simulink model "Assignment1_V4"  (R2022b)
settings: Solver=FixedStepAuto  StartTime=0.0  StopTime=10.0  RelTol=1e-3  EnableMultiTasking=on
undefined symbols (not defined in the file or in its folder): A0, A1, D0, D1, D10, D11, D12, D13, D2, D3, D4, D5, D6, D7, D8, D9, PTA0, PTA1, PTA2, PTB2, PTB23, PTB3, PTB9, PTC16, PTC17, PTC2, PTC3, PTC4, PTD0, PTD1, PTD2, PTD3
libraries: frdmk64flib x25, etargetslib x2
settings Model: ExtModeTrigDuration=5  Creator=a laptop  LastModifiedBy=a laptop
settings OptimizationCC: EnhancedBackFolding=on  PassReuseOutputArgsAs=Individual arguments  ZeroExternalMemoryAtStartup=off  ZeroInternalMemoryAtStartup=off  MaxStackSize=64  OptimizeBlockOrder=speed  DifferentSizesBufferReuse=on  OptimizationCustomize=off  EfficientTunableParamExpr=on
settings DebuggingCC: ParameterTunabilityLossMsg=error
settings HardwareCC: ProdBitPerPointer=32  ProdBitPerSizeT=32  ProdBitPerPtrDiffT=32  ProdLargestAtomicInteger=Long  ProdLargestAtomicFloat=Double  ProdWordSize=32  ProdLongLongMode=on  ProdHWDeviceType=ARM Compatible->ARM Cortex
settings SFSimCC: MATLABDynamicMemAlloc=off
settings RTWCC: Description=Embedded Coder  SystemTargetFile=ert.tlc  HardwareBoard=NXP FRDM-K64F  TLCOptions="-aInlineSetEventsForThisBaseRateFcn=TLC_FALSE -aSuppressMultiTaskScheduler=TLC_FALSE  -aRateBasedStepFcn=0"  TemplateMakefile=ert_default_tmf  Toolchain=GNU Tools for ARM Embedded Processors
settings CodeAppCC: ForceParamTrailComments=on  IgnoreCustomStorageClasses=off  OperatorAnnotations=on  SimulinkDataObjDesc=on  SFDataObjDesc=on  InsertBlockDesc=on
settings ERTTargetCC: SupportVariableSizeSignals=on  ExtModeTransport=4  ExtModeMexFile=sendToCommService

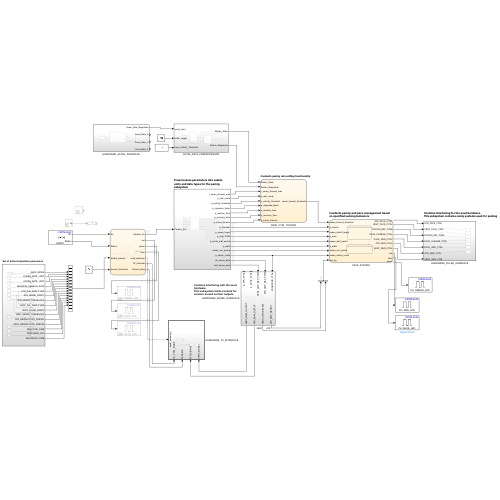
[thumbnail: Simulink's stored preview of the top-level diagram]
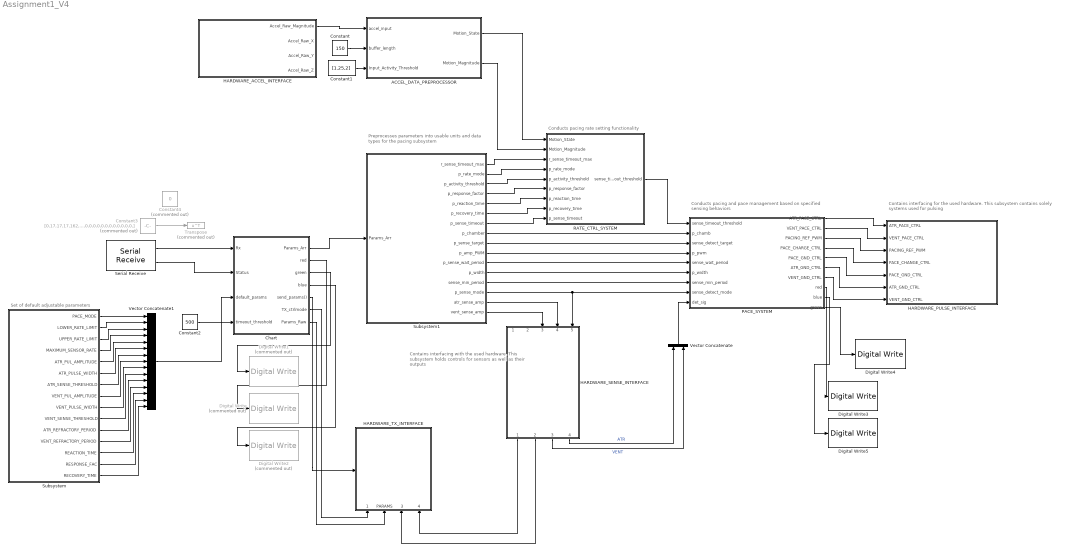
== system Assignment1_V4 ==
  note: Conducts pacing rate setting functionality
  note: Set of default adjustable parameters
  note: Preprocesses parameters into usable units and data types for the pacing subsystem
  note: Contains interfacing with the used hardware.
      | This subsystem holds controls for sensors as well as their outputs
  note: Contains interfacing for the used hardware.
      | This subsystem contains solely systems used for pulsing
  note: Conducts pacing and pace management based on specified sensing behaviors
  ACCEL_DATA_PREPROCESSOR : Subsystem
  Chart : Stateflow chart  TreatAsAtomicUnit=on
      settings: PortSchema="{\"entries\":[{\"content\":{\"sides\":[{\"content\":{\"connectorIds\":[\"In1\",\"In2\",\"In3\",\"In4\"]},\"type\":\"ConnectorPlacement.EquallySpacedRectSide\",\"uuid\":\"320bc760-8283-4f2b-996b-2bacb632d8d9\"},{\"content\":{\"connectorIds\":[\"Out2\",\"Out4\",\"Out5\",\"Out6\",\"Out7\",\"Out3\",\"Out1\"],\"side\":\"RIGHT\"},\"type\":\"ConnectorPlacement.EquallySpacedRectSide\",\"uuid\":\"405a4bb2-50d6-4c0d-b540-a004b1136e76\"},{\"content\":{\"connectorIds\":[],\"side\":\"TOP\"},\"type\":\"ConnectorPlacement.EquallySpacedRectSide\",\"uuid\":\"abc74140-9996-448b-8aab-969529bb67e5\"}]},\"type\":\"ConnectorPlacement.EquallySpacedConnector\",\"uuid\":\"83b64870-f027-44a6-ac9f-b34b790ab38f\"}],\"packageUris\":[\"http://schema.mathworks.com/mf0/Connector/R2020b\"],\"version\":\"1.0\"}"
  Constant : Constant  Value=150
  Constant1 : Constant  Value=[1.25,2]
  Constant2 : Constant  Value=500
  Constant3 : Constant  Commented=on  Value=[0,17,17,17,162,8,0,0,88,2,0,0,176,4,0,0,0,0,0,0,0,0,0,0,0,0,0,0,0,0,0,0,35,0,0,0,10,0,0,0,35,0,0,0,0,0,0,0,128,12,0,0,0,0,0,0,0,0,0,0,0,0,0,0,]  OutDataTypeStr=uint8
  Constant4 : Constant  Commented=on  Value=0  OutDataTypeStr=uint8
  Digital Write : frdmk64flib/Digital Write  Commented=on  Whichpin=RED_LED
  Digital Write1 : frdmk64flib/Digital Write  Commented=on  Whichpin=GREEN_LED
  Digital Write2 : frdmk64flib/Digital Write  Commented=on  Whichpin=BLUE_LED
  Digital Write3 : frdmk64flib/Digital Write  Whichpin=RED_LED
  Digital Write4 : frdmk64flib/Digital Write  Whichpin=GREEN_LED
  Digital Write5 : frdmk64flib/Digital Write  Whichpin=BLUE_LED
  HARDWARE_ACCEL_INTERFACE : Subsystem
  HARDWARE_PULSE_INTERFACE : Subsystem
  HARDWARE_SENSE_INTERFACE : Subsystem
  HARDWARE_TX_INTERFACE : Subsystem
  PACE_SYSTEM : Stateflow chart  TreatAsAtomicUnit=on
      settings: PortSchema="{\"entries\":[{\"content\":{\"sides\":[{\"content\":{\"connectorIds\":[\"In3\",\"In1\",\"In2\",\"In4\",\"In5\",\"In6\",\"In9\",\"In7\",\"In8\"]},\"type\":\"ConnectorPlacement.EquallySpacedRectSide\",\"uuid\":\"7443a3c3-e653-4ca7-8541-eabcfaf454bc\"},{\"content\":{\"connectorIds\":[\"Out1\",\"Out2\",\"Out3\",\"Out4\",\"Out5\",\"Out6\",\"Out7\",\"Out8\",\"Out9\",\"Out10\"],\"side\":\"RIGHT\"},\"type\":\"ConnectorPlacement.EquallySpacedRectSide\",\"uuid\":\"2c63cfa0-dfd9-4a62-91aa-a60ecd75cc2c\"},{\"content\":{\"connectorIds\":[],\"side\":\"TOP\"},\"type\":\"ConnectorPlacement.EquallySpacedRectSide\",\"uuid\":\"5c2dbe0e-7e89-449d-bdd0-c0f7e700edae\"}]},\"type\":\"ConnectorPlacement.EquallySpacedConnector\",\"uuid\":\"602c7a1c-8730-4b31-b945-266bd0371e8b\"}],\"packageUris\":[\"http://schema.mathworks.com/mf0/Connector/R2020b\"],\"version\":\"1.0\"}"
  RATE_CTRL_SYSTEM : Stateflow chart  TreatAsAtomicUnit=on
  Serial Receive : frdmk64flib/Serial Receive  SCIModule=0  Baudrate=uint32(9600)  Parity=None  StopBits=1  HardwareFlowControl=None  ByteOrder=LittleEndian  DataType=uint8  DataLength=64  BlockingMode=off  OutputStatus=on  SampleTime=-1
  Subsystem : Subsystem
  Subsystem1 : Subsystem
  Transpose : Math  Commented=on  Operator=transpose
  Vector Concatenate : Concatenate
  Vector Concatenate1 : Concatenate  NumInputs=15
  wires:
  Serial Receive/2 -> Chart/2(Status)
  RATE_CTRL_SYSTEM/1(sense_timeout_threshold) -> PACE_SYSTEM/3(sense_timeout_threshold)
  Subsystem1/12(p_width) -> PACE_SYSTEM/6(p_width)
  Subsystem/2(LOWER_RATE_LIMIT) -> Vector Concatenate1/2
  Subsystem1/14(p_sense_mode) -> PACE_SYSTEM/7(sense_detect_mode), HARDWARE_SENSE_INTERFACE/5(FRONTEND_CTRL)
  Subsystem1/15(atr_sense_amp) -> HARDWARE_SENSE_INTERFACE/4(ATR_CMP_REF_PWM)
  PACE_SYSTEM/3(PACING_REF_PWM) -> HARDWARE_PULSE_INTERFACE/3(PACING_REF_PWM)
  Chart/6(blue) -> Digital Write2/1
  Chart/5(green) -> Digital Write1/1
  Subsystem1/7(p_sense_timeout) -> RATE_CTRL_SYSTEM/9(p_sense_timeout)
  Constant3/1 -> Transpose/1
  Subsystem1/1(r_sense_timeout_max) -> RATE_CTRL_SYSTEM/3(r_sense_timeout_max)
  Subsystem/13(REACTION_TIME) -> Vector Concatenate1/13
  Subsystem/15(RECOVERY_TIME) -> Vector Concatenate1/15
  HARDWARE_ACCEL_INTERFACE/1(Accel_Raw_Magnitude) -> ACCEL_DATA_PREPROCESSOR/1(accel_input)
  Constant1/1 -> ACCEL_DATA_PREPROCESSOR/3(Input_Activity_Threshold)
  Subsystem/12(VENT_REFRACTORY_PERIOD) -> Vector Concatenate1/12
  Subsystem/10(VENT_SENSE_THRESHOLD) -> Vector Concatenate1/10
  Subsystem1/2(p_rate_mode) -> RATE_CTRL_SYSTEM/4(p_rate_mode)
  Subsystem/6(ATR_PULSE_WIDTH) -> Vector Concatenate1/6
  HARDWARE_SENSE_INTERFACE/2(ATR_RAW_OUTPUT) -> HARDWARE_TX_INTERFACE/3(ATR_SIGNAL)
  Constant2/1 -> Chart/4(timeout_threshold)
  Serial Receive/1 -> Chart/1(Rx)
  Subsystem/8(VENT_PUL_AMPLITUDE) -> Vector Concatenate1/8
  Subsystem1/4(p_response_factor) -> RATE_CTRL_SYSTEM/6(p_response_factor)
  PACE_SYSTEM/5(PACE_GND_CTRL) -> HARDWARE_PULSE_INTERFACE/5(PACE_GND_CTRL)
  PACE_SYSTEM/7(VENT_GND_CTRL) -> HARDWARE_PULSE_INTERFACE/7(VENT_GND_CTRL)
  Subsystem/1(PACE_MODE) -> Vector Concatenate1/1
  Subsystem/3(UPPER_RATE_LIMIT) -> Vector Concatenate1/3
  PACE_SYSTEM/4(PACE_CHARGE_CTRL) -> HARDWARE_PULSE_INTERFACE/4(PACE_CHANGE_CTRL)
  PACE_SYSTEM/6(ATR_GND_CTRL) -> HARDWARE_PULSE_INTERFACE/6(ATR_GND_CTRL)
  Subsystem/5(ATR_PUL_AMPLITUDE) -> Vector Concatenate1/5
  Subsystem1/11(p_sense_wait_period) -> PACE_SYSTEM/5(sense_wait_period)
  Subsystem/9(VENT_PULSE_WIDTH) -> Vector Concatenate1/9
  Subsystem/7(ATR_SENSE_THRESHOLD) -> Vector Concatenate1/7
  Vector Concatenate/1 -> PACE_SYSTEM/8(det_sig)
  Subsystem1/13(sense_min_period) -> PACE_SYSTEM/9(sense_min_period)
  Subsystem1/3(p_activity_threshold) -> RATE_CTRL_SYSTEM/5(p_activity_threshold)
  Subsystem1/5(p_reaction_time) -> RATE_CTRL_SYSTEM/7(p_reaction_time)
  Subsystem/11(ATR_REFRACTORY_PERIOD) -> Vector Concatenate1/11
  Chart/7(send_params()) -> HARDWARE_TX_INTERFACE/Trigger
  Subsystem1/10(p_amp_PWM) -> PACE_SYSTEM/4(p_pwm)
  Subsystem/14(RESPONSE_FAC) -> Vector Concatenate1/14
  Chart/4(red) -> Digital Write/1
  Subsystem1/9(p_sense_target) -> PACE_SYSTEM/2(sense_detect_target)
  Subsystem1/8(p_chamber) -> PACE_SYSTEM/1(p_chamb)
  PACE_SYSTEM/1(ATR_PACE_CTRL) -> HARDWARE_PULSE_INTERFACE/1(ATR_PACE_CTRL)
  HARDWARE_SENSE_INTERFACE/1(VENT_RAW_OUTPUT) -> HARDWARE_TX_INTERFACE/4(VENT_SIGNAL)
  HARDWARE_SENSE_INTERFACE/3(VENT_CMP_DETECT) -> Vector Concatenate/2  "VENT"
  Subsystem1/6(p_recovery_time) -> RATE_CTRL_SYSTEM/8(p_recovery_time)
  ACCEL_DATA_PREPROCESSOR/1(Motion_State) -> RATE_CTRL_SYSTEM/1(Motion_State)
  Chart/3(TX_ctrlmode) -> HARDWARE_TX_INTERFACE/1(TX_CTRL_MODE)
  Vector Concatenate1/1 -> Chart/3(default_params)
  PACE_SYSTEM/2(VENT_PACE_CTRL) -> HARDWARE_PULSE_INTERFACE/2(VENT_PACE_CTRL)
  ACCEL_DATA_PREPROCESSOR/2(Motion_Magnitude) -> RATE_CTRL_SYSTEM/2(Motion_Magnitude)
  Subsystem/4(MAXIMUM_SENSOR_RATE) -> Vector Concatenate1/4
  Chart/1(Params_Raw) -> HARDWARE_TX_INTERFACE/2(PARAMS)
  HARDWARE_SENSE_INTERFACE/4(ATR_CMP_DETECT) -> Vector Concatenate/1  "ATR"
  Constant/1 -> ACCEL_DATA_PREPROCESSOR/2(buffer_length)
  Subsystem1/16(vent_sense_amp) -> HARDWARE_SENSE_INTERFACE/3(VENT_CMP_REF_PWM)
  Chart/2(Params_Arr) -> Subsystem1/1(Params_Arr)
  PACE_SYSTEM/8(red) -> Digital Write3/1
  PACE_SYSTEM/10(green) -> Digital Write4/1
  PACE_SYSTEM/9(blue) -> Digital Write5/1

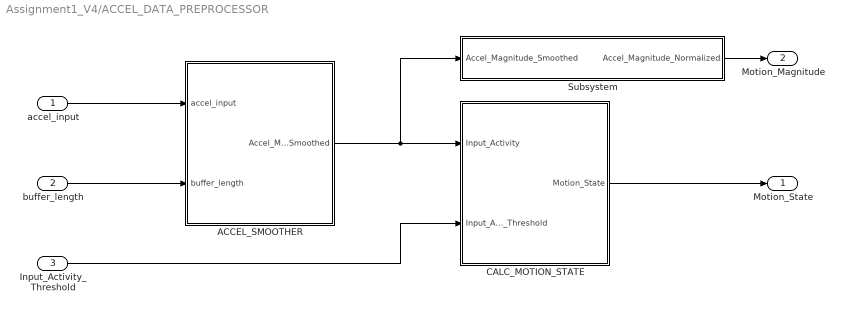
== system Assignment1_V4/ACCEL_DATA_PREPROCESSOR ==
  accel_input : Inport
  buffer_length : Inport  Port=2
  Input_Activity_Threshold : Inport  Port=3
  ACCEL_SMOOTHER : Subsystem
  CALC_MOTION_STATE : Subsystem
  Subsystem : Subsystem
  Motion_State : Outport
  Motion_Magnitude : Outport  Port=2
  wires:
  ACCEL_SMOOTHER/1(Accel_Magnitude_Smoothed) -> Subsystem/1(Accel_Magnitude_Smoothed), CALC_MOTION_STATE/1(Input_Activity)
  accel_input/1 -> ACCEL_SMOOTHER/1(accel_input)
  buffer_length/1 -> ACCEL_SMOOTHER/2(buffer_length)
  CALC_MOTION_STATE/1(Motion_State) -> Motion_State/1
  Input_Activity_Threshold/1 -> CALC_MOTION_STATE/2(Input_Activity_Threshold)
  Subsystem/1(Accel_Magnitude_Normalized) -> Motion_Magnitude/1

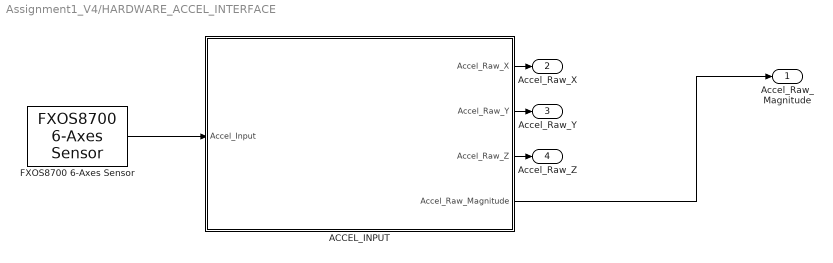
== system Assignment1_V4/HARDWARE_ACCEL_INTERFACE ==
  ACCEL_INPUT : Subsystem
  FXOS8700 6-Axes Sensor : frdmk64flib/FXOS8700 6-Axes Sensor  Activesensor=Accelerometer only  ODR=100Hz  HybridODR=400Hz  Accelfullrange=-4g to +4g  SampleTime=0.01
  Accel_Raw_Magnitude : Outport
  Accel_Raw_X : Outport  Port=2
  Accel_Raw_Y : Outport  Port=3
  Accel_Raw_Z : Outport  Port=4
  wires:
  ACCEL_INPUT/2(Accel_Raw_Y) -> Accel_Raw_Y/1
  ACCEL_INPUT/3(Accel_Raw_Z) -> Accel_Raw_Z/1
  ACCEL_INPUT/1(Accel_Raw_X) -> Accel_Raw_X/1
  FXOS8700 6-Axes Sensor/1 -> ACCEL_INPUT/1(Accel_Input)
  ACCEL_INPUT/4(Accel_Raw_Magnitude) -> Accel_Raw_Magnitude/1

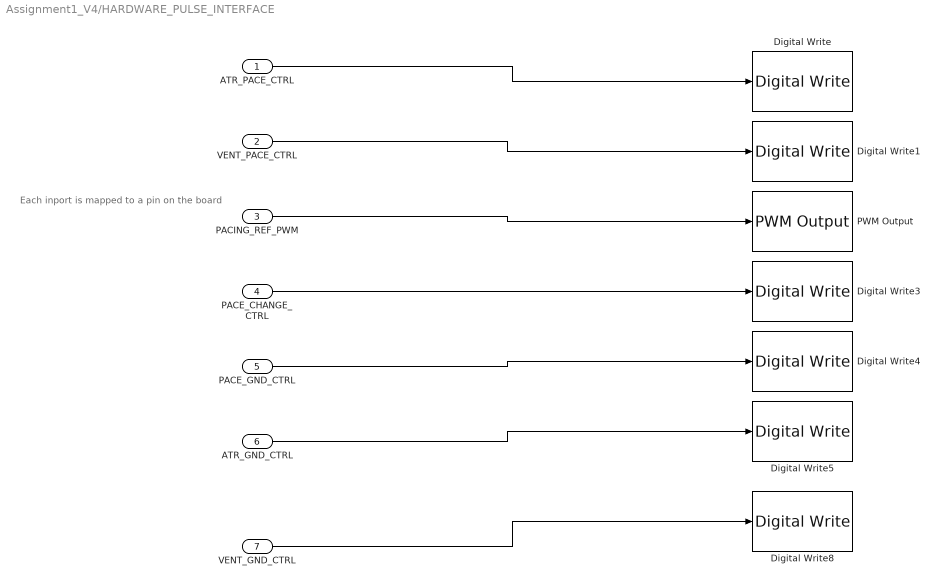
== system Assignment1_V4/HARDWARE_PULSE_INTERFACE ==
  note: Each inport is mapped to a pin on the board
  ATR_PACE_CTRL : Inport
  VENT_PACE_CTRL : Inport  Port=2
  PACING_REF_PWM : Inport  Port=3
  PACE_CHANGE_CTRL : Inport  Port=4
  PACE_GND_CTRL : Inport  Port=5
  ATR_GND_CTRL : Inport  Port=6
  VENT_GND_CTRL : Inport  Port=7
  Digital Write : frdmk64flib/Digital Write  Whichpin=PTA0 (D8)
  Digital Write1 : frdmk64flib/Digital Write  Whichpin=PTC4 (D9)
  Digital Write3 : frdmk64flib/Digital Write  Whichpin=PTB9 (D2)
  Digital Write4 : frdmk64flib/Digital Write  Whichpin=PTD0 (D10)
  Digital Write5 : frdmk64flib/Digital Write  Whichpin=PTD2 (D11)
  Digital Write8 : frdmk64flib/Digital Write  Whichpin=PTD3 (D12)
  PWM Output : frdmk64flib/PWM Output  Whichpin=PTA2 (D5)  InitialFrequency=2000  InitialDutyCycle=0
  wires:
  PACE_CHANGE_CTRL/1 -> Digital Write3/1
  PACE_GND_CTRL/1 -> Digital Write4/1
  VENT_PACE_CTRL/1 -> Digital Write1/1
  VENT_GND_CTRL/1 -> Digital Write8/1
  ATR_PACE_CTRL/1 -> Digital Write/1
  ATR_GND_CTRL/1 -> Digital Write5/1
  PACING_REF_PWM/1 -> PWM Output/1

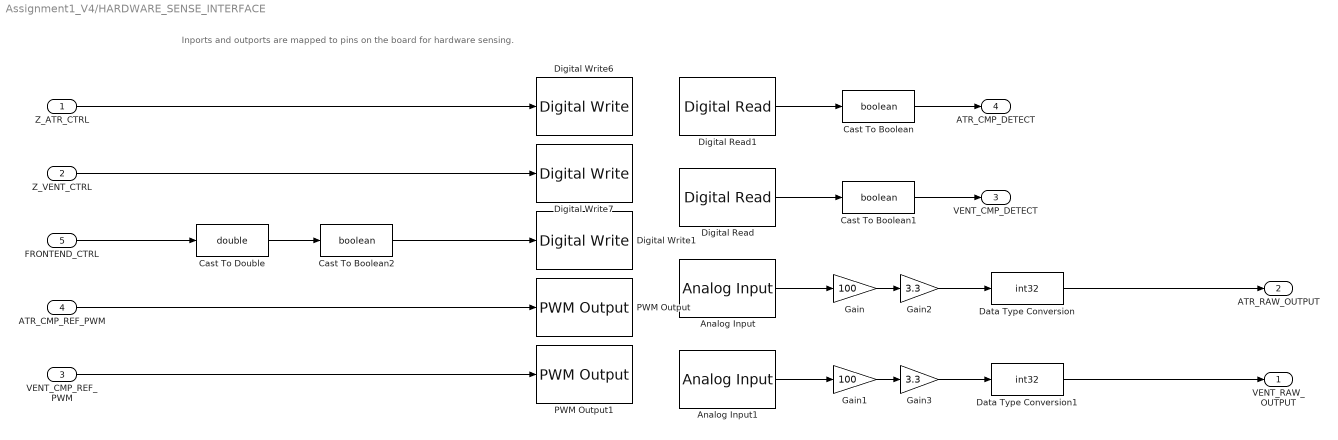
== system Assignment1_V4/HARDWARE_SENSE_INTERFACE ==
  note: Inports and outports are mapped to pins on the board for hardware sensing.
  Z_ATR_CTRL : Inport
  Z_VENT_CTRL : Inport  Port=2
  VENT_CMP_REF_PWM : Inport  Port=3
  ATR_CMP_REF_PWM : Inport  Port=4
  FRONTEND_CTRL : Inport  Port=5
  Analog Input : frdmk64flib/Analog Input  Whichpin=PTB2 (A0)  SampleTime=-1
  Analog Input1 : frdmk64flib/Analog Input  Whichpin=PTB3 (A1)  SampleTime=-1
  Cast To Boolean : DataTypeConversion  OutDataTypeStr=boolean  RndMeth=Round  SaturateOnIntegerOverflow=off
  Cast To Boolean1 : DataTypeConversion  OutDataTypeStr=boolean  RndMeth=Round  SaturateOnIntegerOverflow=off
  Cast To Boolean2 : DataTypeConversion  OutDataTypeStr=boolean  SaturateOnIntegerOverflow=off  RndMeth=Floor
  Cast To Double : DataTypeConversion  OutDataTypeStr=double  SaturateOnIntegerOverflow=off  RndMeth=Floor
  Data Type Conversion : DataTypeConversion  OutDataTypeStr=int32  RndMeth=Floor
  Data Type Conversion1 : DataTypeConversion  OutDataTypeStr=int32  RndMeth=Floor
  Digital Read : frdmk64flib/Digital Read  Whichpin=PTC17 (D1)  SampleTime=0.001
  Digital Read1 : frdmk64flib/Digital Read  Whichpin=PTC16 (D0)  SampleTime=0.001
  Digital Write1 : frdmk64flib/Digital Write  Whichpin=PTD1 (D13)
  Digital Write6 : frdmk64flib/Digital Write  Whichpin=PTB23 (D4)
  Digital Write7 : frdmk64flib/Digital Write  Whichpin=PTC3 (D7)
  Gain : Gain  Gain=100
  Gain1 : Gain  Gain=100
  Gain2 : Gain  Gain=3.3
  Gain3 : Gain  Gain=3.3
  PWM Output : frdmk64flib/PWM Output  Whichpin=PTC2 (D6)  InitialFrequency=2000  InitialDutyCycle=0
  PWM Output1 : frdmk64flib/PWM Output  Whichpin=PTA1 (D3)  InitialFrequency=2000  InitialDutyCycle=0
  VENT_RAW_OUTPUT : Outport
  ATR_RAW_OUTPUT : Outport  Port=2
  VENT_CMP_DETECT : Outport  Port=3
  ATR_CMP_DETECT : Outport  Port=4  OutDataTypeStr=boolean
  wires:
  Z_ATR_CTRL/1 -> Digital Write6/1
  Z_VENT_CTRL/1 -> Digital Write7/1
  FRONTEND_CTRL/1 -> Cast To Double/1
  ATR_CMP_REF_PWM/1 -> PWM Output/1
  VENT_CMP_REF_PWM/1 -> PWM Output1/1
  Digital Read1/1 -> Cast To Boolean/1
  Digital Read/1 -> Cast To Boolean1/1
  Cast To Boolean/1 -> ATR_CMP_DETECT/1
  Cast To Boolean1/1 -> VENT_CMP_DETECT/1
  Cast To Double/1 -> Cast To Boolean2/1
  Cast To Boolean2/1 -> Digital Write1/1
  Analog Input/1 -> Gain/1
  Analog Input1/1 -> Gain1/1
  Gain/1 -> Gain2/1
  Gain1/1 -> Gain3/1
  Data Type Conversion/1 -> ATR_RAW_OUTPUT/1
  Data Type Conversion1/1 -> VENT_RAW_OUTPUT/1
  Gain2/1 -> Data Type Conversion/1
  Gain3/1 -> Data Type Conversion1/1

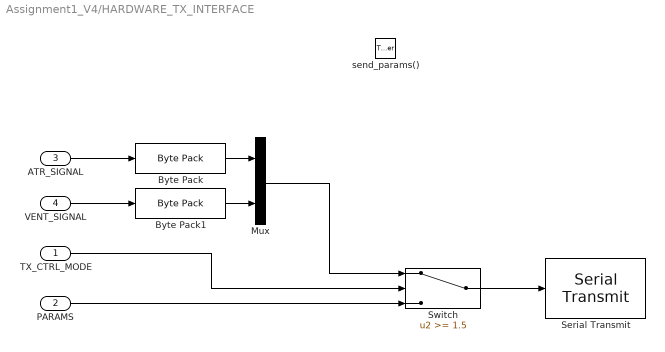
== system Assignment1_V4/HARDWARE_TX_INTERFACE ==
  TX_CTRL_MODE : Inport
  PARAMS : Inport  Port=2  OutDataTypeStr=uint8
  ATR_SIGNAL : Inport  Port=3
  VENT_SIGNAL : Inport  Port=4
  send_params() : TriggerPort  TriggerType=function-call  VariantControl=(inherit)
  Byte Pack : etargetslib/Byte Pack  datatypes={'int32'}  byteAlign=1
  Byte Pack1 : etargetslib/Byte Pack  datatypes={'int32'}  byteAlign=1
  Mux : Mux  Inputs=2
  Serial Transmit : frdmk64flib/Serial Transmit  SCIModule=0  Baudrate=uint32(9600)  Parity=None  StopBits=1  HardwareFlowControl=None  ByteOrder=LittleEndian  BlockingMode=on  OutputStatus=off
  Switch : Switch  Threshold=1.5  OutDataTypeStr=uint8  SaturateOnIntegerOverflow=off  InputSameDT=off
  wires:
  Byte Pack1/1 -> Mux/2
  Byte Pack/1 -> Mux/1
  ATR_SIGNAL/1 -> Byte Pack/1
  VENT_SIGNAL/1 -> Byte Pack1/1
  Switch/1 -> Serial Transmit/1
  Mux/1 -> Switch/1
  TX_CTRL_MODE/1 -> Switch/2
  PARAMS/1 -> Switch/3

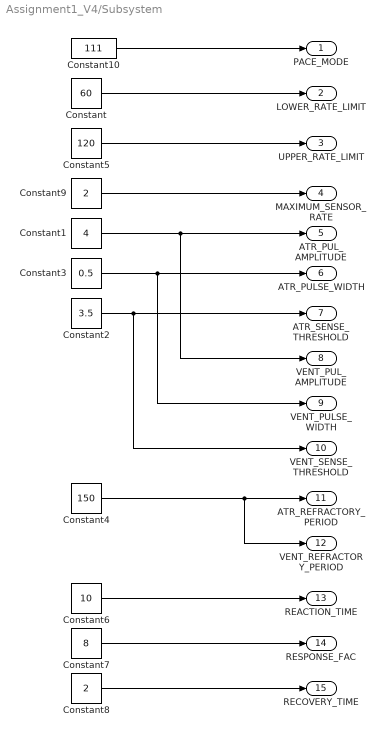
== system Assignment1_V4/Subsystem ==
  Constant : Constant  Value=60
  Constant1 : Constant  Value=4
  Constant10 : Constant  Value=111
  Constant2 : Constant  Value=3.5
  Constant3 : Constant  Value=0.5
  Constant4 : Constant  Value=150
  Constant5 : Constant  Value=120
  Constant6 : Constant  Value=10
  Constant7 : Constant  Value=8
  Constant8 : Constant  Value=2
  Constant9 : Constant  Value=2
  PACE_MODE : Outport
  LOWER_RATE_LIMIT : Outport  Port=2
  UPPER_RATE_LIMIT : Outport  Port=3
  MAXIMUM_SENSOR_RATE : Outport  Port=4
  ATR_PUL_AMPLITUDE : Outport  Port=5
  ATR_PULSE_WIDTH : Outport  Port=6
  ATR_SENSE_THRESHOLD : Outport  Port=7
  VENT_PUL_AMPLITUDE : Outport  Port=8
  VENT_PULSE_WIDTH : Outport  Port=9
  VENT_SENSE_THRESHOLD : Outport  Port=10
  ATR_REFRACTORY_PERIOD : Outport  Port=11
  VENT_REFRACTORY_PERIOD : Outport  Port=12
  REACTION_TIME : Outport  Port=13
  RESPONSE_FAC : Outport  Port=14
  RECOVERY_TIME : Outport  Port=15
  wires:
  Constant10/1 -> PACE_MODE/1
  Constant/1 -> LOWER_RATE_LIMIT/1
  Constant1/1 -> VENT_PUL_AMPLITUDE/1, ATR_PUL_AMPLITUDE/1
  Constant2/1 -> ATR_SENSE_THRESHOLD/1, VENT_SENSE_THRESHOLD/1
  Constant3/1 -> ATR_PULSE_WIDTH/1, VENT_PULSE_WIDTH/1
  Constant4/1 -> VENT_REFRACTORY_PERIOD/1, ATR_REFRACTORY_PERIOD/1
  Constant5/1 -> UPPER_RATE_LIMIT/1
  Constant6/1 -> REACTION_TIME/1
  Constant7/1 -> RESPONSE_FAC/1
  Constant8/1 -> RECOVERY_TIME/1
  Constant9/1 -> MAXIMUM_SENSOR_RATE/1

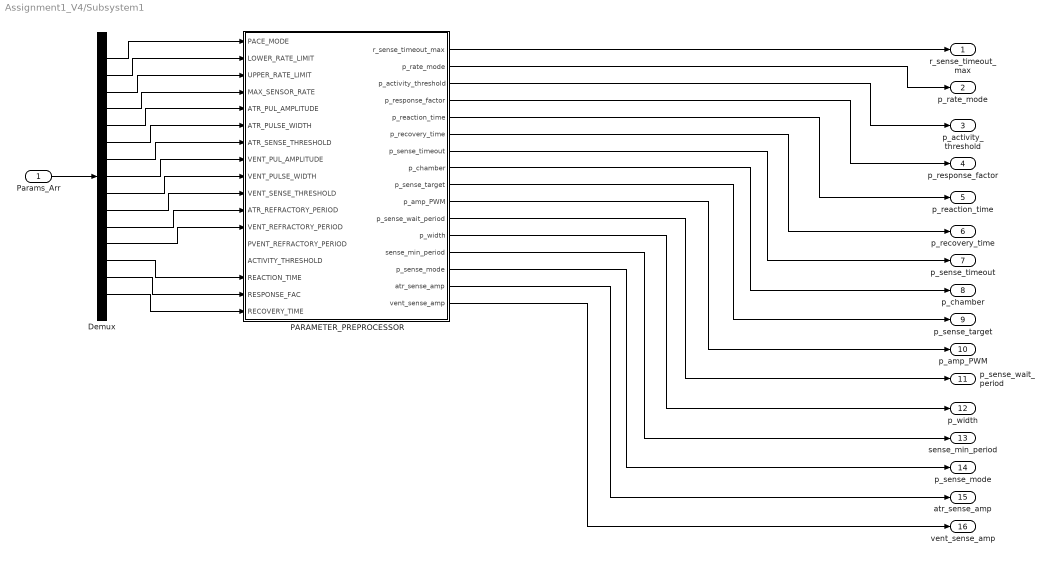
== system Assignment1_V4/Subsystem1 ==
  Params_Arr : Inport
  Demux : Demux  Outputs=15
  PARAMETER_PREPROCESSOR : Subsystem
  r_sense_timeout_max : Outport
  p_rate_mode : Outport  Port=2
  p_activity_threshold : Outport  Port=3
  p_response_factor : Outport  Port=4
  p_reaction_time : Outport  Port=5
  p_recovery_time : Outport  Port=6
  p_sense_timeout : Outport  Port=7
  p_chamber : Outport  Port=8
  p_sense_target : Outport  Port=9
  p_amp_PWM : Outport  Port=10
  p_sense_wait_period : Outport  Port=11
  p_width : Outport  Port=12
  sense_min_period : Outport  Port=13
  p_sense_mode : Outport  Port=14
  atr_sense_amp : Outport  Port=15
  vent_sense_amp : Outport  Port=16
  wires:
  PARAMETER_PREPROCESSOR/11(p_sense_wait_period) -> p_sense_wait_period/1
  PARAMETER_PREPROCESSOR/9(p_sense_target) -> p_sense_target/1
  PARAMETER_PREPROCESSOR/8(p_chamber) -> p_chamber/1
  PARAMETER_PREPROCESSOR/3(p_activity_threshold) -> p_activity_threshold/1
  PARAMETER_PREPROCESSOR/16(vent_sense_amp) -> vent_sense_amp/1
  PARAMETER_PREPROCESSOR/12(p_width) -> p_width/1
  PARAMETER_PREPROCESSOR/15(atr_sense_amp) -> atr_sense_amp/1
  PARAMETER_PREPROCESSOR/14(p_sense_mode) -> p_sense_mode/1
  PARAMETER_PREPROCESSOR/5(p_reaction_time) -> p_reaction_time/1
  PARAMETER_PREPROCESSOR/10(p_amp_PWM) -> p_amp_PWM/1
  PARAMETER_PREPROCESSOR/13(sense_min_period) -> sense_min_period/1
  PARAMETER_PREPROCESSOR/1(r_sense_timeout_max) -> r_sense_timeout_max/1
  PARAMETER_PREPROCESSOR/4(p_response_factor) -> p_response_factor/1
  PARAMETER_PREPROCESSOR/2(p_rate_mode) -> p_rate_mode/1
  PARAMETER_PREPROCESSOR/7(p_sense_timeout) -> p_sense_timeout/1
  PARAMETER_PREPROCESSOR/6(p_recovery_time) -> p_recovery_time/1
  Params_Arr/1 -> Demux/1
  Demux/15 -> PARAMETER_PREPROCESSOR/17(RECOVERY_TIME)
  Demux/14 -> PARAMETER_PREPROCESSOR/16(RESPONSE_FAC)
  Demux/13 -> PARAMETER_PREPROCESSOR/15(REACTION_TIME)
  Demux/12 -> PARAMETER_PREPROCESSOR/12(VENT_REFRACTORY_PERIOD)
  Demux/11 -> PARAMETER_PREPROCESSOR/11(ATR_REFRACTORY_PERIOD)
  Demux/10 -> PARAMETER_PREPROCESSOR/10(VENT_SENSE_THRESHOLD)
  Demux/9 -> PARAMETER_PREPROCESSOR/9(VENT_PULSE_WIDTH)
  Demux/8 -> PARAMETER_PREPROCESSOR/8(VENT_PUL_AMPLITUDE)
  Demux/7 -> PARAMETER_PREPROCESSOR/7(ATR_SENSE_THRESHOLD)
  Demux/6 -> PARAMETER_PREPROCESSOR/6(ATR_PULSE_WIDTH)
  Demux/5 -> PARAMETER_PREPROCESSOR/5(ATR_PUL_AMPLITUDE)
  Demux/4 -> PARAMETER_PREPROCESSOR/4(MAX_SENSOR_RATE)
  Demux/3 -> PARAMETER_PREPROCESSOR/3(UPPER_RATE_LIMIT)
  Demux/2 -> PARAMETER_PREPROCESSOR/2(LOWER_RATE_LIMIT)
  Demux/1 -> PARAMETER_PREPROCESSOR/1(PACE_MODE)

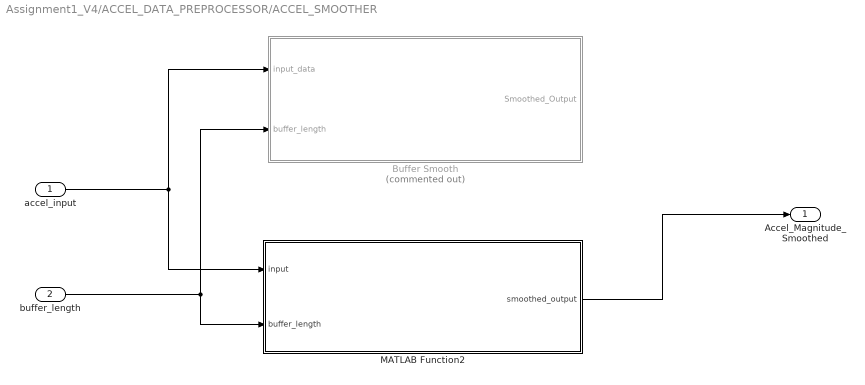
== system Assignment1_V4/ACCEL_DATA_PREPROCESSOR/ACCEL_SMOOTHER ==
  accel_input : Inport
  buffer_length : Inport  Port=2
  Buffer Smooth : Subsystem  Commented=on
  MATLAB Function2 : MATLAB Function  TreatAsAtomicUnit=on
  Accel_Magnitude_Smoothed : Outport
  wires:
  accel_input/1 -> MATLAB Function2/1(input), Buffer Smooth/1(input_data)
  buffer_length/1 -> MATLAB Function2/2(buffer_length), Buffer Smooth/2(buffer_length)
  MATLAB Function2/1(smoothed_output) -> Accel_Magnitude_Smoothed/1

== system Assignment1_V4/ACCEL_DATA_PREPROCESSOR/CALC_MOTION_STATE ==
  Input_Activity : Inport
  Input_Activity_Threshold : Inport  Port=2
  MATLAB Function : MATLAB Function  TreatAsAtomicUnit=on
  Motion_State : Outport
  wires:
  Input_Activity/1 -> MATLAB Function/1(Input_Activity)
  Input_Activity_Threshold/1 -> MATLAB Function/2(Input_Activity_Threshold)
  MATLAB Function/1(Motion_State) -> Motion_State/1

== system Assignment1_V4/ACCEL_DATA_PREPROCESSOR/Subsystem ==
  Accel_Magnitude_Smoothed : Inport
  Gain : Gain  Gain=30
  Accel_Magnitude_Normalized : Outport
  wires:
  Accel_Magnitude_Smoothed/1 -> Gain/1
  Gain/1 -> Accel_Magnitude_Normalized/1

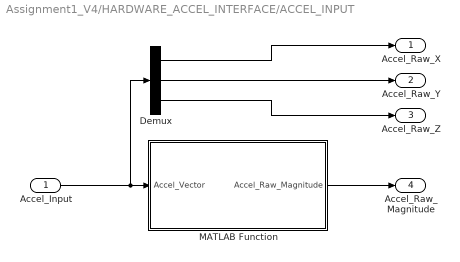
== system Assignment1_V4/HARDWARE_ACCEL_INTERFACE/ACCEL_INPUT ==
  Accel_Input : Inport
  Demux : Demux  Outputs=3
  MATLAB Function : MATLAB Function  TreatAsAtomicUnit=on
  Accel_Raw_X : Outport
  Accel_Raw_Y : Outport  Port=2
  Accel_Raw_Z : Outport  Port=3
  Accel_Raw_Magnitude : Outport  Port=4  OutDataTypeStr=double
  wires:
  Accel_Input/1 -> MATLAB Function/1(Accel_Vector), Demux/1
  Demux/1 -> Accel_Raw_X/1
  Demux/2 -> Accel_Raw_Y/1
  Demux/3 -> Accel_Raw_Z/1
  MATLAB Function/1(Accel_Raw_Magnitude) -> Accel_Raw_Magnitude/1

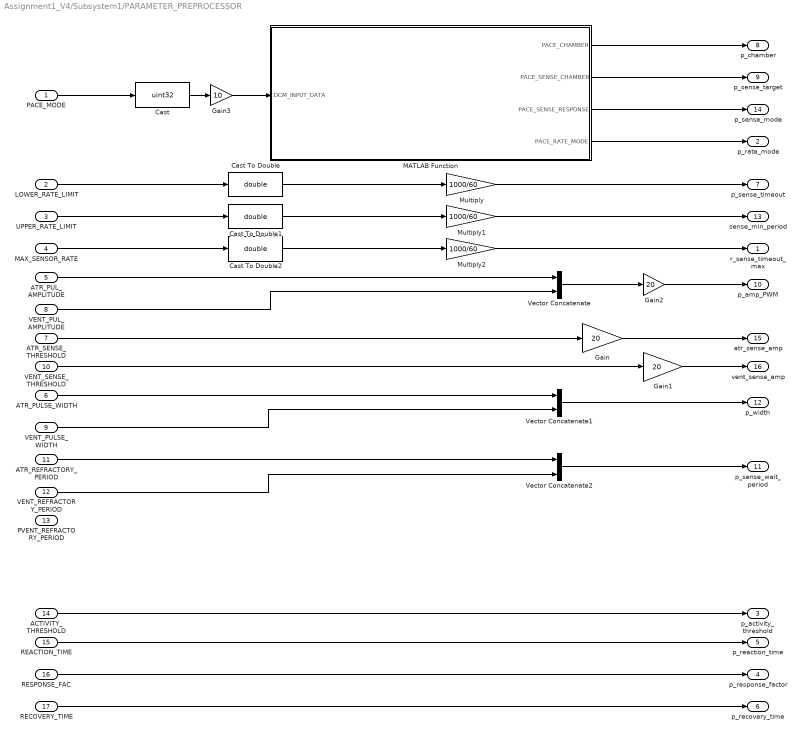
== system Assignment1_V4/Subsystem1/PARAMETER_PREPROCESSOR ==
  PACE_MODE : Inport
  LOWER_RATE_LIMIT : Inport  Port=2
  UPPER_RATE_LIMIT : Inport  Port=3
  MAX_SENSOR_RATE : Inport  Port=4
  ATR_PUL_AMPLITUDE : Inport  Port=5
  ATR_PULSE_WIDTH : Inport  Port=6
  ATR_SENSE_THRESHOLD : Inport  Port=7
  VENT_PUL_AMPLITUDE : Inport  Port=8
  VENT_PULSE_WIDTH : Inport  Port=9
  VENT_SENSE_THRESHOLD : Inport  Port=10
  ATR_REFRACTORY_PERIOD : Inport  Port=11
  VENT_REFRACTORY_PERIOD : Inport  Port=12
  PVENT_REFRACTORY_PERIOD : Inport  Port=13
  ACTIVITY_THRESHOLD : Inport  Port=14
  REACTION_TIME : Inport  Port=15
  RESPONSE_FAC : Inport  Port=16
  RECOVERY_TIME : Inport  Port=17
  Cast : DataTypeConversion  OutDataTypeStr=uint32  RndMeth=Convergent  SaturateOnIntegerOverflow=off
  Cast To Double : DataTypeConversion  OutDataTypeStr=double  SaturateOnIntegerOverflow=off  RndMeth=Floor
  Cast To Double1 : DataTypeConversion  OutDataTypeStr=double  SaturateOnIntegerOverflow=off  RndMeth=Floor
  Cast To Double2 : DataTypeConversion  OutDataTypeStr=double  SaturateOnIntegerOverflow=off  RndMeth=Floor
  Gain : Gain  Gain=20
  Gain1 : Gain  Gain=20
  Gain2 : Gain  Gain=20
  Gain3 : Gain  Gain=10
  MATLAB Function : MATLAB Function  TreatAsAtomicUnit=on
  Multiply : Gain  Gain=1000/60
  Multiply1 : Gain  Gain=1000/60
  Multiply2 : Gain  Gain=1000/60
  Vector Concatenate : Concatenate
  Vector Concatenate1 : Concatenate
  Vector Concatenate2 : Concatenate
  r_sense_timeout_max : Outport
  p_rate_mode : Outport  Port=2
  p_activity_threshold : Outport  Port=3
  p_response_factor : Outport  Port=4
  p_reaction_time : Outport  Port=5
  p_recovery_time : Outport  Port=6
  p_sense_timeout : Outport  Port=7
  p_chamber : Outport  Port=8
  p_sense_target : Outport  Port=9
  p_amp_PWM : Outport  Port=10
  p_sense_wait_period : Outport  Port=11
  p_width : Outport  Port=12
  sense_min_period : Outport  Port=13
  p_sense_mode : Outport  Port=14
  atr_sense_amp : Outport  Port=15
  vent_sense_amp : Outport  Port=16
  wires:
  PACE_MODE/1 -> Cast/1
  MATLAB Function/2(PACE_SENSE_CHAMBER) -> p_sense_target/1
  MATLAB Function/3(PACE_SENSE_RESPONSE) -> p_sense_mode/1
  LOWER_RATE_LIMIT/1 -> Cast To Double/1
  ATR_PUL_AMPLITUDE/1 -> Vector Concatenate/1
  VENT_PUL_AMPLITUDE/1 -> Vector Concatenate/2
  MATLAB Function/1(PACE_CHAMBER) -> p_chamber/1
  ATR_SENSE_THRESHOLD/1 -> Gain/1
  VENT_SENSE_THRESHOLD/1 -> Gain1/1
  Gain2/1 -> p_amp_PWM/1
  Vector Concatenate/1 -> Gain2/1
  ATR_PULSE_WIDTH/1 -> Vector Concatenate1/1
  VENT_PULSE_WIDTH/1 -> Vector Concatenate1/2
  Vector Concatenate1/1 -> p_width/1
  VENT_REFRACTORY_PERIOD/1 -> Vector Concatenate2/2
  Vector Concatenate2/1 -> p_sense_wait_period/1
  ATR_REFRACTORY_PERIOD/1 -> Vector Concatenate2/1
  Cast To Double/1 -> Multiply/1
  Multiply/1 -> p_sense_timeout/1
  Gain1/1 -> vent_sense_amp/1
  Gain/1 -> atr_sense_amp/1
  UPPER_RATE_LIMIT/1 -> Cast To Double1/1
  MAX_SENSOR_RATE/1 -> Cast To Double2/1
  MATLAB Function/4(PACE_RATE_MODE) -> p_rate_mode/1
  RECOVERY_TIME/1 -> p_recovery_time/1
  RESPONSE_FAC/1 -> p_response_factor/1
  REACTION_TIME/1 -> p_reaction_time/1
  ACTIVITY_THRESHOLD/1 -> p_activity_threshold/1
  Multiply1/1 -> sense_min_period/1
  Cast To Double1/1 -> Multiply1/1
  Multiply2/1 -> r_sense_timeout_max/1
  Cast To Double2/1 -> Multiply2/1
  Cast/1 -> Gain3/1
  Gain3/1 -> MATLAB Function/1(DCM_INPUT_DATA)

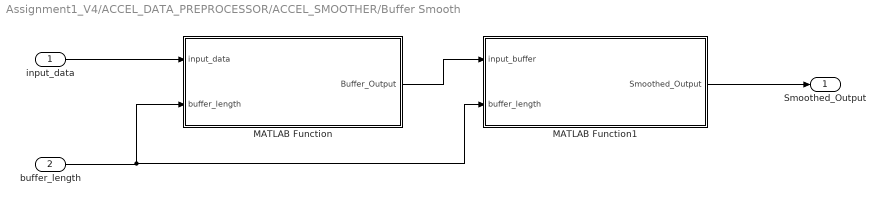
== system Assignment1_V4/ACCEL_DATA_PREPROCESSOR/ACCEL_SMOOTHER/Buffer Smooth ==
  input_data : Inport
  buffer_length : Inport  Port=2  OutMin=1  OutMax=1000
  MATLAB Function : MATLAB Function  TreatAsAtomicUnit=on
  MATLAB Function1 : MATLAB Function  TreatAsAtomicUnit=on
  Smoothed_Output : Outport
  wires:
  input_data/1 -> MATLAB Function/1(input_data)
  MATLAB Function1/1(Smoothed_Output) -> Smoothed_Output/1
  buffer_length/1 -> MATLAB Function1/2(buffer_length), MATLAB Function/2(buffer_length)
  MATLAB Function/1(Buffer_Output) -> MATLAB Function1/1(input_buffer)

== matlab function Assignment1_V4/HARDWARE_ACCEL_INTERFACE/ACCEL_INPUT/MATLAB Function ==
  data: Accel_Vector input; Accel_Raw_Magnitude output
function Accel_Raw_Magnitude = Get_Magnitude(Accel_Vector)
    Accel_Raw_Magnitude = (Accel_Vector(1)^2 + Accel_Vector(2)^2 + Accel_Vector(3)^2)^(1/2);
end

== matlab function Assignment1_V4/Subsystem1/PARAMETER_PREPROCESSOR/MATLAB Function ==
  data: DCM_INPUT_DATA input; PACE_CHAMBER output Enum: Pace_Chamber; PACE_SENSE_CHAMBER output Enum: Pace_Sense_Chamber; PACE_SENSE_RESPONSE output Enum: Pace_Sense_Response; PACE_RATE_MODE output Enum: Pace_Rate_Mode
function [PACE_CHAMBER, PACE_SENSE_CHAMBER, PACE_SENSE_RESPONSE, PACE_RATE_MODE] = Decode_Pacemode(DCM_INPUT_DATA)
   % disp(DCM_INPUT_DATA)
    PACE_CHAMBER = Pace_Chamber(parse(DCM_INPUT_DATA,3));
    PACE_SENSE_CHAMBER = Pace_Sense_Chamber(parse(DCM_INPUT_DATA,2));
    PACE_SENSE_RESPONSE = Pace_Sense_Response(parse(DCM_INPUT_DATA,1));
    PACE_RATE_MODE = Pace_Rate_Mode(parse(DCM_INPUT_DATA,0));
end

function output = parse(DCM_INPUT_DATA, Bit_Depth)
    output = round((mod(double(DCM_INPUT_DATA), 10^(Bit_Depth+1)) - mod(double(DCM_INPUT_DATA), 10^Bit_Depth))/(10^Bit_Depth));
end

== stateflow chart Assignment1_V4/PACE_SYSTEM ==
  note: PACE sends pulses to the specified body part
  state PACE
    state Charge
      %Stop discharge of C22
      PACE_GND_CTRL = true;
      VENT_PACE_CTRL = false;
      ATR_PACE_CTRL = false;
      %Discharge blocking capacitor
      if p_chamb == Pace_Chamber.Atrium
      ATR_GND_CTRL = true;
      VENT_GND_CTRL = false;
      else
      ATR_GND_CTRL = false;
      VENT_GND_CTRL = true;
      end
      %Charge C22
      ATR_PACE_CTRL = false;
      VENT_PACE_CTRL = false;
      PACING_REF_PWM = p_pwm(double(p_chamb));
      PACE_CHARGE_CTRL = true;
      send(pace_compl)
    state Discharge_Prep
      %Prepares discharge
      %Stop charging C22
      PACING_REF_PWM = 0;
      PACE_CHARGE_CTRL = false;
      PACE_GND_CTRL = true;
      %Stop discharging blocking capacitor
      ATR_GND_CTRL = false;
      VENT_GND_CTRL = false;
    state Pace_Atr
      ATR_PACE_CTRL = true;
    state Pace_Vent
      VENT_PACE_CTRL = true;
    (default) -> Discharge_Prep
    Pace_Atr -> Charge : after(p_width(double(p_chamb)), msec)
    Discharge_Prep -> Pace_Atr [order 1] : [p_chamb == Pace_Chamber.Atrium]
    Discharge_Prep -> Pace_Vent [order 2] : [p_chamb == Pace_Chamber.Ventricle]
    Pace_Vent -> Charge : after(p_width(double(p_chamb)), msec)
  state SENSE
    state Sense_Finish
    state Sense_Disabled
      %All sensor timing is disabled
    state Sense_Wait
      %Sensor prep
      red  = 1;
      green = 0;
      blue = 0;
    note: Warm-up period before sensor is active
    state Sense_Fail
      red = 0;
      green = 0;
      blue = 0;
      %Starts the pacing process
      send(sense_timeout);
    state Sense_Detect
      %Sensor active period
      red = 0;
      green = 1;
      blue = 0;
    state Sense_Detected
      red = 0;
      green = 0;
      blue = 0;
    note: This state is present for future DCM interactions and data logging
    (default) -> Sense_Finish
    Sense_Finish -> Sense_Disabled [order 2] : [sense_detect_mode == Pace_Sense_Response.Nothing]
    Sense_Finish -> Sense_Wait [order 1] : [sense_detect_mode ~= Pace_Sense_Response.Nothing]
    Sense_Disabled -> Sense_Fail : after(sense_timeout_threshold, msec)
    Sense_Detected -> Sense_Wait
    Sense_Wait -> Sense_Detect : after(sense_wait_period(double(sense_detect_target)), msec)
    Sense_Detect -> Sense_Fail [order 1] : [after(sense_timeout_threshold - sense_wait_period(double(sense_detect_target)), msec)]
    Sense_Detect -> Sense_Detected [order 2] : [det_sig(double(sense_detect_target)) == true]
  note: SENSE conducts all timing related operations and activates PACE when needed
  SENSE -> PACE : sense_timeout
  PACE -> SENSE : pace_compl
  (default) -> SENSE
  data: p_chamb input Enum: Pace_Chamber; sense_detect_target input; sense_timeout_threshold input double; p_pwm input; sense_wait_period input double; ATR_PACE_CTRL output; VENT_PACE_CTRL output; PACING_REF_PWM output; PACE_CHARGE_CTRL output; PACE_GND_CTRL output; ATR_GND_CTRL output; VENT_GND_CTRL output; p_width input double; sense_detect_mode input Enum: Pace_Sense_Response; det_sig input; sense_min_period input; red output; blue output; green output
  events: sense_timeout local FUNCTION_CALL_EVENT; pace_compl local FUNCTION_CALL_EVENT

== matlab function Assignment1_V4/ACCEL_DATA_PREPROCESSOR/ACCEL_SMOOTHER/Buffer Smooth/MATLAB Function ==
  data: input_data input; Buffer_Output output; buffer_length input
function Buffer_Output = Generate_Buffer(input_data, buffer_length)
    persistent Buffer_Internal;
    if (isempty(Buffer_Internal))
        Buffer_Internal = ones(50); %upper bound 1000
    else
        for i = 1:buffer_length-1
            Buffer_Internal(buffer_length-i+1) = Buffer_Internal(buffer_length-i);
        end
        Buffer_Internal(1) = input_data;
    end
    Buffer_Output = Buffer_Internal;
end

== matlab function Assignment1_V4/ACCEL_DATA_PREPROCESSOR/ACCEL_SMOOTHER/Buffer Smooth/MATLAB Function1 ==
  data: input_buffer input; Smoothed_Output output; buffer_length input
function Smoothed_Output = Smooth_Output(input_buffer, buffer_length)
    Sum_Value = 0;
    for i = 1:buffer_length
        Sum_Value = Sum_Value + input_buffer(i);
    end
    Smoothed_Output = Sum_Value/buffer_length;
end

== matlab function Assignment1_V4/ACCEL_DATA_PREPROCESSOR/CALC_MOTION_STATE/MATLAB Function ==
  data: Input_Activity input; Motion_State output; Input_Activity_Threshold input
function Motion_State = Determine_Motion_State(Input_Activity, Input_Activity_Threshold)
    Motion_State_num = 3;
    for i = 2:-1:1
         if Input_Activity_Threshold(i) > Input_Activity
               Motion_State_num = i;
         end
    end
    Motion_State = Motion_State_num;
end

== stateflow chart Assignment1_V4/Chart ==
  state Save_Buf_Params
    entry:
    Params_Arr = Output_Candidate;
    green = 1;
  state Init
    entry:
    Params_Arr = default_params;
    Output_Candidate = default_params
    Params_Raw = ones(8,1,'uint8');
  state ECG_TX_Loop_Standby
    entry:
    TX_ctrlmode = 2;
    send_params();
    %red = 1;
    %green = 0;
    %blue = 0;
  state Detect_Cur_Mode
    entry:
    Rx_buf = Rx;
    Op_Mode = uint32(typecast(Rx_buf(1:4), 'uint32'));
    TX_ctrlmode = 1;
    red = 0;
    green = 0;
    blue = 0;
  state Conv_Data
    entry:
    Output_Candidate = Process_Rx(Rx_buf(5:end));
    %Params_Arr = Process_Rx(Rx_buf(5:end)); %TEST
    Rxint_buf = reshape(Rx_buf, 8,8);
    iter = 1;
  state TX_Rxint_buf
    entry:
    Params_Raw = uint8(Rxint_buf(:,iter));
    send_params();
    iter = iter+1;
  state TX_wait
    entry:
    blue = 1
  Save_Buf_Params -> ECG_TX_Loop_Standby : [after(20,msec)]
  Detect_Cur_Mode -> Save_Buf_Params [order 1] : [Op_Mode == hex2dec('11111111')]
  Detect_Cur_Mode -> ECG_TX_Loop_Standby [order 3] : [Op_Mode ~= hex2dec('11111100') & Op_Mode ~= hex2dec('11111111')]
  (default) -> Init
  ECG_TX_Loop_Standby -> ECG_TX_Loop_Standby [order 2] : [after(7,msec)]
  Detect_Cur_Mode -> Conv_Data [order 2] : [Op_Mode == hex2dec('11111100')]
  Init -> ECG_TX_Loop_Standby
  ECG_TX_Loop_Standby -> Detect_Cur_Mode [order 1] : [Status == 0]
  TX_wait -> ECG_TX_Loop_Standby [order 2] : [after(timeout_threshold, msec)]
  TX_wait -> Detect_Cur_Mode [order 1] : [Status == 0]
  TX_Rxint_buf -> Detect_Cur_Mode [order 2] : [Status == 0]
  Conv_Data -> TX_Rxint_buf
  TX_Rxint_buf -> TX_Rxint_buf [order 3] : [after(10,msec)]
  TX_Rxint_buf -> TX_wait [order 1] : [iter >= 9]
  data: Rx_input function_input; output_set function_output; Rx input uint8; Status input uint8; Output_Candidate local double; Params_Raw output uint8; Op_Mode local uint32; default_params input double; timeout_threshold input double; Params_Arr output double; TX_ctrlmode output uint8; iter local uint8; Rxint_buf local uint8; Rx_buf local; red output; green output; blue output
  events: send_params output FUNCTION_CALL_EVENT
  function output_set = Process_Rx(Rx_input):
    | function output_set = Process_Rx(Rx_input)
    |     output_set = zeros(15,1,'double');
    |     for i = 1:15
    |         tmp = typecast(Rx_input(1+(i-1)*4 : i*4),'uint32');
    |         output_set(i) = double(tmp)/10;
    |     end
    | end

== matlab function Assignment1_V4/ACCEL_DATA_PREPROCESSOR/ACCEL_SMOOTHER/MATLAB Function2 ==
  data: input input; smoothed_output output; buffer_length input
function smoothed_output = rolling_average_smooth(input, buffer_length)
    persistent rolling_avg;
    persistent init_counter;

    if (isempty(init_counter)) 
        init_counter = 0; 
        rolling_avg = 0;
    end

    if (init_counter < buffer_length)
        init_counter = init_counter + 1;
    end
    rolling_avg = rolling_avg * (init_counter-1)/(init_counter) + input/init_counter;

    smoothed_output = rolling_avg;
end

== stateflow chart Assignment1_V4/RATE_CTRL_SYSTEM ==
  state Init
    sense_timeout_threshold = p_sense_timeout;
  state Calc_Init_Params [commented out]
  state ? [commented out]
    state Check_Activity [commented out]
    state Raise_Pace [commented out]
    state Reduce_Pace [commented out]
    (default) -> Check_Activity [commented out]
    Check_Activity -> Raise_Pace [commented out] : [Motion_State == Rate_Motion_State.High]
    Check_Activity -> Reduce_Pace [commented out] : [Motion_State ~= Rate_Motion_State.High]
  (default) -> Init
  data: Motion_State input; Motion_Magnitude input; r_sense_timeout_max input; p_rate_mode input; p_activity_threshold input; p_response_factor input; p_reaction_time input; p_recovery_time input; sense_timeout_threshold output; p_sense_timeout input
